simulink model "CelsiustoFahrenheit"  (R2015a)
settings: Solver=ode45  StartTime=0.0  StopTime=1000  RelTol=1e-3
settings Model: Creator=John  LastModifiedBy=John
settings DataIOCC: ExternalInput=[t,tempC]  LoadExternalInput=on  SignalLoggingSaveFormat=ModelDataLogs

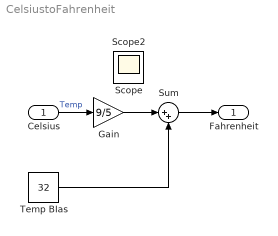
== system CelsiustoFahrenheit ==
  "Celsius " : Inport
  Gain : Gain  Gain=9/5
  Sum : Sum  Inputs=|++
  "Temp BIas " : Constant  Value=32
  "Fahrenheit " : Outport
  Scope : Scope
  Scope2 : Scope
      settings: SaveName=ScopeData2
  wires:
  "Temp BIas "/1 -> Sum/2
  "Celsius "/1 -> Gain/1  "Temp"
  Gain/1 -> Sum/1
  Sum/1 -> "Fahrenheit "/1
